simulink model "KF_3_gdl_AHRS_Dataset2"  (R2020b)
settings: Solver=FixedStepAuto  StartTime=0.0  StopTime=1000  FixedStep=1/200  RelTol=1e-3
values from neighbouring files (symbols this model uses):
  BARO_cov = single(1.7)/2    [init_1gdl.m]    (also in init_3_gdl_AHRS_fb.m = single(1.7)/5; init_3gdl.m; init_dati_veri.m = single(1.7)/5)
  BARO_cov_old = single(1.7)/2    [init_1gdl.m]    (also in init_3_gdl_AHRS_fb.m; init_3gdl.m; init_dati_veri.m)
  bj_x = 0.4    [init_3_gdl_AHRS_fb.m]
  bj_y = 0.9    [init_3_gdl_AHRS_fb.m]
  bj_z = 0.5    [init_3_gdl_AHRS_fb.m]
  bjy = bj_y - 0.1    (= 0.8)    [init_3_gdl_AHRS_fb.m]
  filter_pos = tf(1,[1 1])    [init_1gdl.m]    (also in init_3_gdl_AHRS_fb.m; init_3gdl.m; init_dati_veri.m)
  filter_pos_Z = tf(1,[0.5 1])    [init_3_gdl_AHRS_fb.m]    (also in init_3gdl.m; init_dati_veri.m)
  g_ned = [0; 0; -9.81]    [init_3_gdl_AHRS_fb.m]    (also in init_dati_veri.m)
  GPS_cov = single([1*2, 1])/2    [init_1gdl.m]    (also in init_3_gdl_AHRS_fb.m = single([0.1*50, 0.1*50, 200*5, 200*5, 0.36])/2; init_3gdl.m = single([1*2, 1*2, 1, 1, 0.36])/2; init_dati_veri.m = single([0.1, 0.1, 200*5, 200*5, 0.36])/2)
  GPS_cov_old = single([0.1, 0.1, 200, 200, 0.36])/2    [init_1gdl.m]    (also in init_3_gdl_AHRS_fb.m = single([0.1, 0.1, 200, 200, 0.36]/2); init_3gdl.m; init_dati_veri.m = single([0.1, 0.1, 200, 200, 0.36]/2))
  IMU_cov = single(15*0.07)/2    [init_1gdl.m]    (also in init_3_gdl_AHRS_fb.m = single([15*[0.07*50, 0.07*50] 15*50*0.09])/2; init_3gdl.m = single([15*[0.07, 0.07] 10*0.09])/2; init_dati_veri.m = single([15*[0.07*5, 0.07*5] 15*50*0.09])/2)
  IMU_cov_old = single([15*[0.07, 0.07] 10*0.09])/2    [init_1gdl.m]    (also in init_3_gdl_AHRS_fb.m = single([15*[0.07, 0.07] 10*0.09]/2); init_3gdl.m; init_dati_veri.m = single([15*[0.07, 0.07] 10*0.09]/2))
  Q = single(diag([1e-2, 1e-6, 1e-4, 1e-12]))*2    [init_1gdl.m]    (also in init_3_gdl_AHRS_fb.m = single(diag([px,vx,ax,py,vy,ay,pz,vz,az,bx,by,bz]))*2; init_3gdl.m = single(diag([px,vx,ax,py,vy,ay,pz,vz,az,bx,by,bz]))*2; init_dati_veri.m = single(diag([px,vx,ax,py,vy,ay,pz,vz,az,bx,by,bz]))*2)
  Q_old = single(diag([1e-8, 1e-1, 1e-2, 1e-8, 1e-1, 1e-2, 1e-5, 1e-4, 0.010]))*2    [init_1gdl.m]    (also in init_3_gdl_AHRS_fb.m; init_3gdl.m; init_dati_veri.m)
  ST = 1/200    (= 0.005)    [init_1gdl.m]    (also in init_3_gdl_AHRS_fb.m; init_3gdl.m; init_dati_veri.m)
  T_50 = 1/50    (= 0.02)    [init_1gdl.m]    (also in init_3_gdl_AHRS_fb.m; init_3gdl.m; init_dati_veri.m)
  var_giroscopio = [(deg2rad(0.16))^2;(deg2rad(0.16))^2;(deg2rad(0.16))^2]    [init_3_gdl_AHRS_fb.m]    (also in init_dati_veri.m)
  var_p_x = 2    [init_3_gdl_AHRS_fb.m]    (also in init_3gdl.m = 1; init_dati_veri.m)
  var_p_y = 2    [init_3_gdl_AHRS_fb.m]    (also in init_3gdl.m = 1; init_dati_veri.m)
  var_p_z = 0.30    (= 0.3)    [init_3_gdl_AHRS_fb.m]    (also in init_3gdl.m = 0.15; init_dati_veri.m)
  var_v_x = 0.60    (= 0.6)    [init_3_gdl_AHRS_fb.m]    (also in init_3gdl.m = 0.3; init_dati_veri.m)
  var_v_y = 0.32    [init_3_gdl_AHRS_fb.m]    (also in init_3gdl.m = 0.16; init_dati_veri.m)
  var_v_z = 0.60    (= 0.6)    [init_3_gdl_AHRS_fb.m]    (also in init_3gdl.m = 0.3; init_dati_veri.m)
undefined symbols (not defined in the file or in its folder): DiscIntNeverNeededParam
libraries: simulink x33, cstblocks x9
(part 1 of 4)
settings Model: Creator=chiara-s  LastModifiedBy=chiara-s

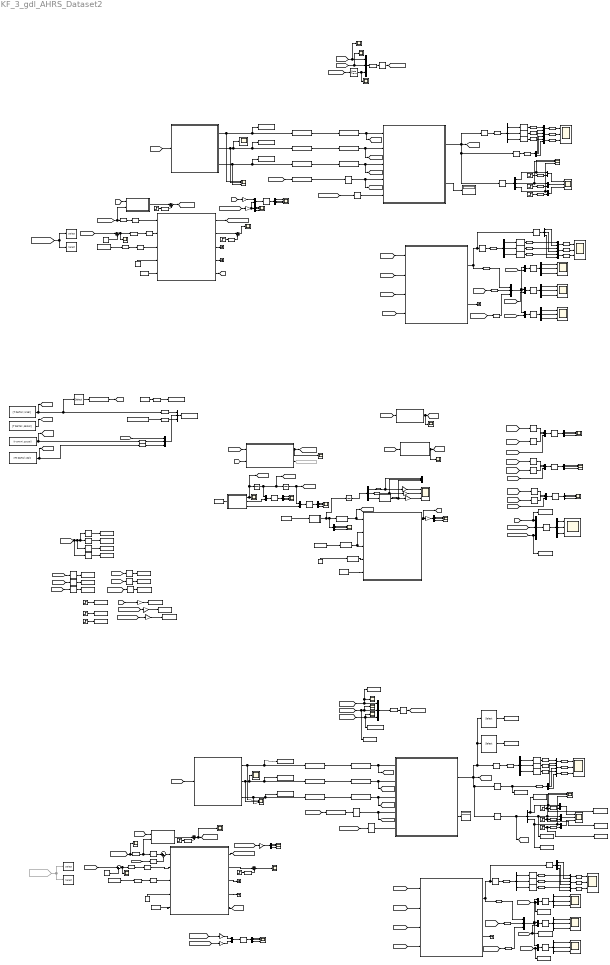
== system KF_3_gdl_AHRS_Dataset2 ==
  note: confronto filtro con feedback e filtro senza
  note: NO BIAS FEEDBACK
  note: AHRS CON FEEDBACK BIAS
  note: misurement DATA (già in NED)
  note: TAKE DATA
  note: inertial data
  note: KF_a_bordo_DATA
  note: FLAGS
  ACC : Scope  NumInputPorts=3
  ACC confronto : Scope  NumInputPorts=3
  ACC1 : Scope  NumInputPorts=3
  ACC_AHRS_NED1 : Scope
  ACC_DOPO_AHRS_NED COMPENSATO DI GRAVITA' : Scope
  ACC_DOPO_AHRS_NED COMPENSATO DI GRAVITA'1 : Scope
  CONFRONTO BIAS : Scope  NumInputPorts=3
  CONFRONTO BIAS1 : Scope  NumInputPorts=3
  Cast To Single{,1..5} (6 alike) : DataTypeConversion  OutDataTypeStr=single
  Confronto RPY_conRPY_feedback : Scope  NumInputPorts=3
  Constant : Constant  Value=[0;0;0]  VectorParams1D=off
  Constant1 : Constant  Value=[0;0;0]
  DATASET NOSTRO1 : MATLAB Function  TreatAsAtomicUnit=on
  Data Type Conversion{1..51,53,67..75,77..89} (74 alike) : DataTypeConversion  OutDataTypeStr=single
  Demux{,1..2,4..6,10..12,16,21..23,31,36} (15 alike) : Demux  Outputs=3
  Demux{13..14,19..20} (4 alike) : Demux  Outputs=[2 2 2]
  Demux{3,15,17..18} (4 alike) : Demux  Outputs=[3 3 3]
  Demux{7..9,37..39} (6 alike) : Demux  Outputs=[4 4 4]
  Digital Clock : DigitalClock  SampleTime=0.005
  Digital Clock1 : DigitalClock  SampleTime=0.02
  Digital Clock2 : DigitalClock  SampleTime=1/200
  Discrete Derivative{,1..11} (12 alike) : simulink/Discrete/Discrete Derivative  gainval=1.0  ICPrevScaledInput=0.0  OutMin=[]  OutMax=[]  OutDataType=fixdt(1, 16)  OutScaling=2^-10  DoSatur=off
  Discrete-Time Integrator : DiscreteIntegrator  SampleTime=-1  ICPrevOutput=DiscIntNeverNeededParam  ICPrevScaledInput=DiscIntNeverNeededParam
  Discrete-Time Integrator1 : DiscreteIntegrator  SampleTime=-1  ICPrevOutput=DiscIntNeverNeededParam  ICPrevScaledInput=DiscIntNeverNeededParam
  Discrete-Time Integrator2 : DiscreteIntegrator  SampleTime=-1  ICPrevOutput=DiscIntNeverNeededParam  ICPrevScaledInput=DiscIntNeverNeededParam
  Display : Display
  Display1 : Display
  Dpos VS vel_stima{,1..3} (4 alike) : Scope  NumInputPorts=3
  FLAG : Scope  NumInputPorts=3
  FLAG1 : Scope  NumInputPorts=3
  Flag computation : MATLAB Function  TreatAsAtomicUnit=on
  Flag computation1 : MATLAB Function  TreatAsAtomicUnit=on
  From73 : From  Commented=on  GotoTag=inertial_data
  Gain{,1..8,18..20} (12 alike) : Gain  Gain=180/pi
  Goto11 : Goto  Commented=on  GotoTag=accelorometro_vero
  MATLAB Function : MATLAB Function  TreatAsAtomicUnit=on
  MATLAB Function1 : MATLAB Function  TreatAsAtomicUnit=on
  MATLAB Function2 : MATLAB Function  TreatAsAtomicUnit=on
  MATLAB Function3 : MATLAB Function  TreatAsAtomicUnit=on
  MPU AHRS1 : Subsystem
  MPU AHRS3 : Subsystem
  MPU AHRS4 : Subsystem
  Mux{,1..5,8,11,13..19,24..25,27,37,39..43,46,56,63..64} (28 alike) : Mux  Inputs=2
  Mux{6..7,9..10,12,20..23,26,67} (11 alike) : Mux  Inputs=3
  Navigation Filter SINGLE 50 Hz NOSTRO : MATLAB Function  TreatAsAtomicUnit=on  mask{Q=Q, GPS_cov=GPS_cov, IMU_cov=IMU_cov, BARO_cov=BARO_cov}
      mask prompts: Q "Q matrix"; GPS_cov "R matrix - GPS covariance [px py vx vy vz]"; IMU_cov "R matrix - IMU covariance [ax ay az]"; BARO_cov "R matrix - BARO covariance"
  Navigation Filter SINGLE 50 Hz NOSTRO1 : MATLAB Function  TreatAsAtomicUnit=on  mask{Q=Q, GPS_cov=GPS_cov, IMU_cov=IMU_cov, BARO_cov=BARO_cov}
      mask prompts: Q "Q matrix"; GPS_cov "R matrix - GPS covariance [px py vx vy vz]"; IMU_cov "R matrix - IMU covariance [ax ay az]"; BARO_cov "R matrix - BARO covariance"
  Navigation Filter SINGLE 50 Hz1 : MATLAB Function  TreatAsAtomicUnit=on  mask{Q=Q_old, GPS_cov=GPS_cov, IMU_cov=IMU_cov, BARO_cov=BARO_cov}
      mask prompts: Q "Q matrix"; GPS_cov "R matrix - GPS covariance [px py vx vy vz]"; IMU_cov "R matrix - IMU covariance [ax ay az]"; BARO_cov "R matrix - BARO covariance"
  Navigation Filter SINGLE 50 Hz2 : MATLAB Function  TreatAsAtomicUnit=on  mask{Q=Q_old, GPS_cov=GPS_cov_old, IMU_cov=IMU_cov_old, BARO_cov=BARO_cov_old}
      mask prompts: Q "Q matrix"; GPS_cov "R matrix - GPS covariance [px py vx vy vz]"; IMU_cov "R matrix - IMU covariance [ax ay az]"; BARO_cov "R matrix - BARO covariance"
  POS confronto : Scope  NumInputPorts=3
  POSITION : Scope  NumInputPorts=3
  POSITION1 : Scope  NumInputPorts=3
  RPY : Scope  NumInputPorts=3
  RPY degree : Scope  NumInputPorts=3
  RPY degree2 : Scope  NumInputPorts=3
  RPY1 : Scope  NumInputPorts=3
  Random Number : RandomNumber  Variance=var_giroscopio  Seed=[1; 5; 3]  SampleTime=1/200  VectorParams1D=off
  Random Number1 : RandomNumber  Variance=var_giroscopio  Seed=[1; 5; 3]  SampleTime=1/200  VectorParams1D=off
  Rate Transition{1,3..4,11,15,30..35} (11 alike) : RateTransition  OutPortSampleTime=1/50
  Rate Transition{5..8,16..18} (7 alike) : RateTransition  OutPortSampleTime=1/200
  Scope{,4..6} (4 alike) : Scope  NumInputPorts=3
  Scope1 : Scope
  Scope2 : Scope
  Scope7 : Scope
  Selector : Selector  InputPortWidth=12  IndexOptions=Index vector (dialog)  Indices=[10 11 12]  OutputSizes=1
  Selector{1,5,19..20,33,47} (6 alike) : Selector  InputPortWidth=12  IndexOptions=Index vector (dialog)  Indices=[1 4 7]  OutputSizes=1
  Selector10 : Selector  InputPortWidth=30+3  IndexOptions=Index vector (dialog)  Indices=[2 11 23 31 5 14 26 32 8 17 29 33]  OutputSizes=1
  Selector11 : Selector  InputPortWidth=30+3  IndexOptions=Index vector (dialog)  Indices=[3 12 24 31 6 15 27 32 9 18 30 33]  OutputSizes=1
  Selector12 : Selector  InputPortWidth=9  IndexOptions=Index vector (dialog)  Indices=[1 4 7]  OutputSizes=1
  Selector13 : Selector  InputPortWidth=30+3  IndexOptions=Index vector (dialog)  Indices=[1 10 22 31 4 13 25 32 7 16 28 33]  OutputSizes=1
  Selector14 : Selector  InputPortWidth=9  IndexOptions=Index vector (dialog)  Indices=[2 5 8]  OutputSizes=1
  Selector15 : Selector  InputPortWidth=9  IndexOptions=Index vector (dialog)  Indices=[2 5 8]  OutputSizes=1
  Selector{16..17,28,30} (4 alike) : Selector  InputPortWidth=6  IndexOptions=Index vector (dialog)  Indices=[1 4 2 5 3 6]  OutputSizes=1
  Selector{2,18,21,24,27,31} (6 alike) : Selector  InputPortWidth=9  IndexOptions=Index vector (dialog)  Indices=[1 4 7 2 5 8 3 6 9]  OutputSizes=1
  Selector{3,22..23,29,46} (5 alike) : Selector  InputPortWidth=12  IndexOptions=Index vector (dialog)  Indices=[2 5 8]  OutputSizes=1
  Selector{25..26,32,48} (4 alike) : Selector  InputPortWidth=12  IndexOptions=Index vector (dialog)  Indices=[3 6 9]  OutputSizes=1
  Selector4 : Selector  InputPortWidth=12  IndexOptions=Index vector (dialog)  Indices=[10 11 12]  OutputSizes=1
  Selector49 : Selector  InputPortWidth=12  IndexOptions=Index vector (dialog)  Indices=[10 11 12]  OutputSizes=1
  Selector6 : Selector  InputPortWidth=30+3  IndexOptions=Index vector (dialog)  Indices=[2 11 23 31 5 14 26 32 8 17 29 33]  OutputSizes=1
  Selector7 : Selector  InputPortWidth=30+3  IndexOptions=Index vector (dialog)  Indices=[3 12 24 31 6 15 27 32 9 18 30 33]  OutputSizes=1
  Selector8 : Selector  InputPortWidth=9  IndexOptions=Index vector (dialog)  Indices=[1 4 7]  OutputSizes=1
  Selector9 : Selector  InputPortWidth=30+3  IndexOptions=Index vector (dialog)  Indices=[1 10 22 31 4 13 25 32 7 16 28 33]  OutputSizes=1
  Subsystem : Subsystem
  Subsystem1 : Subsystem
  Subsystem2 : Subsystem
  Sum{,1,3..6} (6 alike) : Sum  Inputs=|++
  Sum2 : Sum  Inputs=|+-
  Terminator{,1..5} (6 alike) : Terminator
  To Workspace : ToWorkspace  VariableName=pos_vera  SaveFormat=Timeseries  SampleTime=-1
  To Workspace1 : ToWorkspace  VariableName=vel_vera  SaveFormat=Timeseries  SampleTime=-1
  To Workspace10 : ToWorkspace  VariableName=baro_fix_flag  SampleTime=-1
  To Workspace11 : ToWorkspace  VariableName=acc_misura  SaveFormat=Timeseries  SampleTime=-1
  To Workspace12 : ToWorkspace  VariableName=vel_misura  SaveFormat=Timeseries  SampleTime=-1
  To Workspace13 : ToWorkspace  VariableName=pos_misura  SaveFormat=Timeseries  SampleTime=-1
  To Workspace14 : ToWorkspace  VariableName=bias_x  SaveFormat=Timeseries  SampleTime=-1
  To Workspace15 : ToWorkspace  VariableName=bias_y  SaveFormat=Timeseries  SampleTime=-1
  To Workspace16 : ToWorkspace  VariableName=bias_z  SaveFormat=Timeseries  SampleTime=-1
  To Workspace17 : ToWorkspace  VariableName=vel_stima  SaveFormat=Timeseries  SampleTime=-1
  To Workspace18 : ToWorkspace  VariableName=acc_stima  SaveFormat=Timeseries  SampleTime=-1
  To Workspace19 : ToWorkspace  VariableName=rpy_vera  SaveFormat=Timeseries  SampleTime=-1
  To Workspace2 : ToWorkspace  VariableName=acc_vera  SaveFormat=Timeseries  SampleTime=-1
  To Workspace20 : ToWorkspace  VariableName=rpy_feedback  SaveFormat=Timeseries  SampleTime=-1
  To Workspace21 : ToWorkspace  VariableName=pos_stima  SaveFormat=Timeseries  SampleTime=-1
  To Workspace22 : ToWorkspace  VariableName=bx_cost  SaveFormat=Timeseries  SampleTime=-1
  To Workspace23 : ToWorkspace  VariableName=by_cost  SaveFormat=Timeseries  SampleTime=-1
  To Workspace24 : ToWorkspace  VariableName=bz_cost  SaveFormat=Timeseries  SampleTime=-1
  To Workspace3 : ToWorkspace  VariableName=gps_fix_flag  SampleTime=-1
  To Workspace4 : ToWorkspace  VariableName=init_flag  SampleTime=-1
  To Workspace5 : ToWorkspace  VariableName=DATA_1  SampleTime=-1
  To Workspace6 : ToWorkspace  VariableName=T_1  SampleTime=-1
  To Workspace7 : ToWorkspace  VariableName=gps_fix_flag1  SampleTime=-1
  To Workspace73 : ToWorkspace  VariableName=pos_misura1  SaveFormat=Timeseries  SampleTime=-1
  To Workspace74 : ToWorkspace  VariableName=vel_misura1  SaveFormat=Timeseries  SampleTime=-1
  To Workspace75 : ToWorkspace  VariableName=pos_vera1  SaveFormat=Timeseries  SampleTime=-1
  To Workspace76 : ToWorkspace  VariableName=vel_vera1  SaveFormat=Timeseries  SampleTime=-1
  To Workspace77 : ToWorkspace  VariableName=acc_vera1  SaveFormat=Timeseries  SampleTime=-1
  To Workspace78 : ToWorkspace  VariableName=pos_stima1  SaveFormat=Timeseries  SampleTime=-1
  To Workspace79 : ToWorkspace  VariableName=vel_stima1  SaveFormat=Timeseries  SampleTime=-1
  To Workspace8 : ToWorkspace  VariableName=init_flag1  SampleTime=-1
  To Workspace80 : ToWorkspace  VariableName=acc_stima1  SaveFormat=Timeseries  SampleTime=-1
  To Workspace81 : ToWorkspace  VariableName=bias_stima1  SaveFormat=Timeseries  SampleTime=-1
  To Workspace82 : ToWorkspace  VariableName=bx_vero  SaveFormat=Timeseries  SampleTime=-1
  To Workspace83 : ToWorkspace  VariableName=by_vero  SaveFormat=Timeseries  SampleTime=-1
  To Workspace84 : ToWorkspace  VariableName=acc_misura1  SaveFormat=Timeseries  SampleTime=-1
  To Workspace85 : ToWorkspace  VariableName=bz_vero  SaveFormat=Timeseries  SampleTime=-1
  To Workspace86 : ToWorkspace  VariableName=rpy_ideali  SaveFormat=Timeseries  SampleTime=-1
  To Workspace87 : ToWorkspace  VariableName=rpy  SaveFormat=Timeseries  SampleTime=-1
  To Workspace88 : ToWorkspace  VariableName=rpy_fb  SaveFormat=Timeseries  SampleTime=-1
  To Workspace9 : ToWorkspace  VariableName=baro_fix_flag1  SampleTime=-1
  VEL confronto : Scope  NumInputPorts=3
  VELOCITY : Scope  NumInputPorts=3
  VELOCITY1 : Scope  NumInputPorts=3
  acc : Scope
  acc_body_g : Scope
  acccc2 : Scope
  acccc3 : Scope
  angular rate : Scope  NumInputPorts=3
  b_x : Step  Time=0  After=bj_x  SampleTime=T_50
  b_x1 : Step  Time=0  After=bj_x  SampleTime=T_50
  b_x5 : Step  Time=0  After=bj_x  SampleTime=T_50
  b_y : Step  Time=0  After=bj_y  SampleTime=T_50
  b_y1 : Step  Time=0  After=bjy  SampleTime=T_50
  b_y5 : Step  Time=0  After=bjy  SampleTime=T_50
  b_z : Step  Time=0  After=bj_z  SampleTime=T_50
  b_z1 : Step  Time=0  After=bj_z  SampleTime=T_50
  b_z5 : Step  Time=0  After=bj_z  SampleTime=T_50
  disable1 : Constant  Value=0
  disable2 : Constant  Value=0
  disable3 : Constant  Value=0
  dummy VICON angles 1 : Constant  Value=[0; 0; 0]  OutDataTypeStr=single
  dummy VICON angles 2 : Constant  Value=[0; 0; 0]  OutDataTypeStr=single
  dummy VICON angles 3 : Constant  Value=[0; 0; 0]  OutDataTypeStr=single
  get MAG1 : Selector  InputPortWidth=15  IndexOptions=Index vector (dialog)  Indices=[11:13]  OutputSizes=1
  get MAG2 : Selector  InputPortWidth=15  IndexOptions=Index vector (dialog)  Indices=[5:7]  OutputSizes=1
  get MAG3 : Selector  InputPortWidth=15  IndexOptions=Index vector (dialog)  Indices=[11:13]  OutputSizes=1
  get OMEGA4 : Selector  InputPortWidth=15  IndexOptions=Index vector (dialog)  Indices=[5:7]  OutputSizes=1
  get RPY1 : Selector  InputPortWidth=15  IndexOptions=Index vector (dialog)  Indices=[2:4]  OutputSizes=1
  get flags 1 : FromWorkspace  VariableName=[Tt DATA(:,34)]  SampleTime=0.02  OutputAfterFinalValue=Holding final value
  "get measurement data " : FromWorkspace  VariableName=[T DATA(:,25:33)]  SampleTime=0.02  OutputAfterFinalValue=Holding final value
  get navdata(KF) : FromWorkspace  VariableName=[T DATA(:,16:24)]  SampleTime=0.02  OutputAfterFinalValue=Holding final value
  get navdata4 : FromWorkspace  VariableName=[T DATA(:,1:15)]  SampleTime=0.02  Interpolate=off  OutputAfterFinalValue=Holding final value
  get navdata5 : FromWorkspace  VariableName=[T DATA(:,35:40)]  SampleTime=0.02  Interpolate=off  OutputAfterFinalValue=Holding final value
  gps fix1 : Scope
  gps fix2 : Scope
  gravity : Step  Time=0  After=[0; 0; 9.81]  SampleTime=1/200
  gravity1 : Step  Time=11.02  After=[0; 0; 9.81]  SampleTime=1/200
  gravity2 : Step  Time=0  After=[0; 0; 9.81]  SampleTime=1/200
  gravity3 : Step  Time=0  After=[0; 0; 9.81]  SampleTime=1/200
  mag : Constant  Value=[0;0;0]
  pos : Scope  NumInputPorts=3
  pos_misura : Scope
  poss2 : Scope
  poss3 : Scope
  vel : Scope  NumInputPorts=3
  vel_misura : Scope
  velll2 : Scope
  velll3 : Scope
  wires:
  Data Type Conversion19/1 -> To Workspace6/1
  Data Type Conversion25/1 -> Data Type Conversion26/1
  Data Type Conversion17/1 -> Mux10/1
  Data Type Conversion29/1 -> Rate Transition4/1
  [x_out_filter] -> Mux12/1
  Data Type Conversion28/1 -> [flag_baro], Navigation Filter SINGLE 50 Hz NOSTRO/3(flagBARO)
  Navigation Filter SINGLE 50 Hz NOSTRO/1(xout) -> Selector/1, Selector3/1, [x_out_filter], Selector1/1
  get navdata4/1 -> get RPY1/1, Data Type Conversion17/1, [inertial_data]
  Data Type Conversion18/1 -> Mux12/2
  Data Type Conversion24/1 -> [flag_init_ok], Navigation Filter SINGLE 50 Hz NOSTRO/1(flagINITOK)
  Mux12/1 -> Mux10/2
  Data Type Conversion22/1 -> Mux10/3
  Data Type Conversion27/1 -> Data Type Conversion28/1
  Flag computation/1(init) -> To Workspace8/1, Data Type Conversion23/1, FLAG/1
  Data Type Conversion21/1 -> Mux12/3
  get navdata5/1 -> Data Type Conversion22/1
  Digital Clock1/1 -> Data Type Conversion19/1
  Navigation Filter SINGLE 50 Hz NOSTRO/2(Pout) -> Display/1
  Data Type Conversion26/1 -> [flag_GPS], Navigation Filter SINGLE 50 Hz NOSTRO/2(flagGPS)
  get flags 1/1 -> [flag_data], Data Type Conversion21/1
  Rate Transition4/1 -> [measure], Navigation Filter SINGLE 50 Hz NOSTRO/4(measure)
  Data Type Conversion23/1 -> Data Type Conversion24/1
  Flag computation/2(gps) -> To Workspace7/1, Data Type Conversion25/1, gps fix1/1, FLAG/2
  "get measurement data "/1 -> [measurements], Data Type Conversion18/1
  get navdata(KF)/1 -> [nav_data_KF]
  Flag computation/3(baro) -> To Workspace9/1, Data Type Conversion27/1, FLAG/3
  Mux10/1 -> To Workspace5/1
  Selector1/1 -> Data Type Conversion13/1
  [dataset_AHRS] -> Data Type Conversion29/1
  Selector/1 -> Demux1/1
  b_x/1 -> Data Type Conversion3/1
  Mux/1 -> CONFRONTO BIAS/1
  Demux1/2 -> Scope/2, Mux2/1
  b_y/1 -> Data Type Conversion2/1
  Mux2/1 -> CONFRONTO BIAS/2
  b_z/1 -> Data Type Conversion1/1
  Demux1/3 -> Scope/3, Mux1/1
  Mux1/1 -> CONFRONTO BIAS/3
  Data Type Conversion1/1 -> Mux1/2
  Data Type Conversion2/1 -> Mux2/2
  Demux/1 -> Discrete Derivative/1
  Demux/2 -> Discrete Derivative2/1
  Demux/3 -> Discrete Derivative1/1
  Selector3/1 -> Data Type Conversion14/1
  Mux3/1 -> Data Type Conversion32/1
  Demux2/1 -> Mux3/2
  Mux4/1 -> Data Type Conversion31/1
  Demux2/2 -> Mux4/2
  Mux5/1 -> Data Type Conversion30/1
  Demux2/3 -> Mux5/2
  Data Type Conversion13/1 -> Demux/1
  Data Type Conversion14/1 -> Demux2/1
  Discrete Derivative1/1 -> Data Type Conversion15/1
  Data Type Conversion15/1 -> Mux5/1
  Discrete Derivative2/1 -> Data Type Conversion16/1
  Data Type Conversion16/1 -> Mux4/1
  Discrete Derivative/1 -> Data Type Conversion20/1
  Data Type Conversion20/1 -> Mux3/1
  Data Type Conversion30/1 -> Dpos VS vel_stima/3
  Data Type Conversion31/1 -> Dpos VS vel_stima/2
  Data Type Conversion32/1 -> Dpos VS vel_stima/1
  Data Type Conversion3/1 -> Mux/2
  Demux1/1 -> Scope/1, Mux/1
  get RPY1/1 -> Data Type Conversion33/1
  Data Type Conversion33/1 -> [RPY]
  [RPY_AHRS] -> Rate Transition1/1
  Demux6/1 -> RPY degree/1
  Demux6/2 -> RPY degree/2
  Demux6/3 -> RPY degree/3
  [flag_init_ok] -> Navigation Filter SINGLE 50 Hz1/1(flagINITOK)
  [flag_GPS] -> Navigation Filter SINGLE 50 Hz1/2(flagGPS)
  [flag_baro] -> Navigation Filter SINGLE 50 Hz1/3(flagBARO)
  [measure] -> Navigation Filter SINGLE 50 Hz1/4(measure)
  Navigation Filter SINGLE 50 Hz1/2(Pout) -> Terminator/1
  Navigation Filter SINGLE 50 Hz1/1(xout) -> Data Type Conversion34/1, Selector14/1, Selector12/1
  [x_out_filter] -> Data Type Conversion35/1
  [dataset_AHRS] -> Data Type Conversion36/1
  Data Type Conversion34/1 -> Mux9/1
  Data Type Conversion35/1 -> Mux9/2
  Data Type Conversion36/1 -> Mux9/3
  Selector13/1 -> Demux7/1
  Demux7/1 -> POSITION/1
  Demux7/2 -> POSITION/2
  Demux7/3 -> POSITION/3
  Selector10/1 -> Demux8/1
  Selector11/1 -> Demux9/1
  Demux9/1 -> ACC/1
  Demux9/2 -> ACC/2
  Demux9/3 -> ACC/3
  Demux8/1 -> VELOCITY/1
  Demux8/2 -> VELOCITY/2
  Demux8/3 -> VELOCITY/3
  Discrete Derivative4/1 -> Data Type Conversion38/1
  Data Type Conversion37/1 -> Demux10/1
  Demux10/1 -> Discrete Derivative3/1
  Discrete Derivative3/1 -> Data Type Conversion40/1
  Discrete Derivative5/1 -> Data Type Conversion39/1
  Demux10/2 -> Discrete Derivative5/1
  Demux10/3 -> Discrete Derivative4/1
  Selector12/1 -> Data Type Conversion37/1
  Data Type Conversion40/1 -> Mux11/1
  Mux14/1 -> Data Type Conversion41/1
  Data Type Conversion39/1 -> Mux13/1
  Data Type Conversion41/1 -> Dpos VS vel_stima1/3
  Data Type Conversion38/1 -> Mux14/1
  Mux13/1 -> Data Type Conversion42/1
  Data Type Conversion42/1 -> Dpos VS vel_stima1/2
  Mux11/1 -> Data Type Conversion43/1
  Data Type Conversion43/1 -> Dpos VS vel_stima1/1
  Selector14/1 -> Demux11/1
  Demux11/1 -> Mux11/2
  Demux11/2 -> Mux13/2
  Demux11/3 -> Mux14/2
  Mux15/1 -> Selector13/1
  Mux16/1 -> Selector10/1
  Mux17/1 -> Selector11/1
  Mux9/1 -> Mux17/1, Mux15/1, Mux16/1
  [pos_ned_vera] -> Mux15/2
  [vel_ned_vera] -> Mux16/2
  [acc_ned_vera] -> Mux17/2
  disable1/1 -> MPU AHRS1/4(vicon_enable)
  Data Type Conversion45/1 -> Rate Transition6/1
  Rate Transition6/1 -> MPU AHRS1/3(MAG)
  Data Type Conversion44/1 -> Rate Transition5/1
  Rate Transition7/1 -> MPU AHRS1/2(PQR)
  dummy VICON angles 1/1 -> MPU AHRS1/5(Vicon_ori)
  MPU AHRS1/1(RPY_MPU) -> [RPY_AHRS]
  MPU AHRS1/4(debiased PQR) -> Terminator1/1
  MPU AHRS1/3(filter running) -> Terminator2/1
  [inertial_data] -> get MAG1/1, get MAG2/1
  Data Type Conversion46/1 -> Rate Transition7/1
  [RPY_AHRS] -> Gain/1
  Rate Transition1/1 -> Navigation Filter SINGLE 50 Hz NOSTRO/5(euler_in)
  MPU AHRS1/5(Rt) -> [Rt]
  Rate Transition11/1 -> Navigation Filter SINGLE 50 Hz NOSTRO1/5(euler_in)
  Data Type Conversion8/1 -> Mux63/1
  Demux22/3 -> Discrete Derivative10/1
  Data Type Conversion69/1 -> Data Type Conversion70/1
  [RPY_AHRS_fd] -> Rate Transition11/1
  MPU AHRS4/5(Rt) -> [Rt_fd]
  Demux23/2 -> Mux39/2
  MPU AHRS4/2(ACC_NED) -> Sum3/1
  Flag computation1/1(init) -> FLAG1/1, To Workspace4/1, Data Type Conversion51/1
  Selector4/1 -> [bias_stima_fd], Demux16/1
  Mux37/1 -> Data Type Conversion86/1
  MPU AHRS4/4(debiased PQR) -> Terminator4/1
  MPU AHRS4/3(filter running) -> Terminator5/1
  Selector8/1 -> Data Type Conversion80/1
  Data Type Conversion84/1 -> Dpos VS vel_stima3/3
  Demux36/3 -> RPY degree2/3
  Demux39/1 -> ACC1/1
  Data Type Conversion48/1 -> Mux56/1
  Mux41/1 -> Selector9/1
  Mux39/1 -> Data Type Conversion85/1
  Selector9/1 -> Demux37/1
  Data Type Conversion5/1 -> Demux5/1
  Gain5/1 -> Demux36/1
  Flag computation1/2(gps) -> gps fix2/1, To Workspace3/1, Data Type Conversion67/1, FLAG1/2
  Selector7/1 -> Demux39/1
  Data Type Conversion78/1 -> Mux67/2
  Navigation Filter SINGLE 50 Hz NOSTRO1/2(Pout) -> Display1/1
  Mux56/1 -> Data Type Conversion75/1
  Mux63/1 -> Data Type Conversion74/1
  Data Type Conversion83/1 -> Mux37/1
  Discrete Derivative6/1 -> Data Type Conversion48/1
  [x_out_filter_fd] -> Data Type Conversion78/1
  From73/1 -> get MAG3/1, get OMEGA4/1
  Navigation Filter SINGLE 50 Hz2/2(Pout) -> Terminator3/1
  dummy VICON angles 2/1 -> MPU AHRS4/5(Vicon_ori)
  Mux67/1 -> Mux43/1, Mux41/1, Mux42/1
  Data Type Conversion89/1 -> Rate Transition18/1
  MPU AHRS4/1(RPY_MPU) -> [RPY_AHRS_fd]
  [RPY_AHRS_fd] -> Gain5/1
  Demux16/1 -> To Workspace14/1, Scope5/1, Mux8/1
  Demux37/3 -> POSITION1/3
  Mux43/1 -> Selector7/1
  disable2/1 -> MPU AHRS4/4(vicon_enable)
  Rate Transition17/1 -> MPU AHRS4/3(MAG)
  Rate Transition18/1 -> MPU AHRS4/2(PQR)
  Discrete Derivative11/1 -> Data Type Conversion82/1
  [pos_ned_vera] -> To Workspace/1, Mux41/2
  Data Type Conversion80/1 -> Demux22/1
  [flag_GPS_fd] -> Navigation Filter SINGLE 50 Hz2/2(flagGPS)
  Selector15/1 -> Demux23/1
  Mux46/1 -> CONFRONTO BIAS1/2
  Demux38/1 -> VELOCITY1/1
  Data Type Conversion85/1 -> Dpos VS vel_stima3/2
  Data Type Conversion74/1 -> Dpos VS vel_stima2/2
  Demux38/3 -> VELOCITY1/3
  Demux22/1 -> Discrete Derivative9/1
  Data Type Conversion82/1 -> Mux39/1
  Mux42/1 -> Selector6/1
  Discrete Derivative9/1 -> Data Type Conversion83/1
  Demux23/1 -> Mux37/2
  Rate Transition15/1 -> [measure_fd], Navigation Filter SINGLE 50 Hz NOSTRO1/4(measure)
  Demux22/2 -> Discrete Derivative11/1
  Data Type Conversion81/1 -> Mux40/1
  Discrete Derivative10/1 -> Data Type Conversion81/1
  Demux38/2 -> VELOCITY1/2
  Demux39/3 -> ACC1/3
  Demux39/2 -> ACC1/2
  Data Type Conversion67/1 -> Data Type Conversion68/1
  Discrete Derivative7/1 -> Data Type Conversion7/1
  Selector6/1 -> Demux38/1
  Demux37/2 -> POSITION1/2
  Data Type Conversion77/1 -> Mux67/1
  Data Type Conversion79/1 -> Mux67/3
  Demux36/2 -> RPY degree2/2
  Data Type Conversion75/1 -> Dpos VS vel_stima2/1
  Demux36/1 -> RPY degree2/1
  Selector29/1 -> To Workspace17/1, Data Type Conversion6/1
  Demux31/2 -> Mux63/2
  Demux31/3 -> Mux64/2
  b_z1/1 -> To Workspace24/1, Data Type Conversion4/1
  b_y1/1 -> To Workspace23/1, Data Type Conversion12/1
  Data Type Conversion12/1 -> Mux46/2
  Data Type Conversion4/1 -> Mux27/2
  [dataset_AHRS_fd] -> Data Type Conversion79/1
  Data Type Conversion70/1 -> [flag_baro_fd], Navigation Filter SINGLE 50 Hz NOSTRO1/3(flagBARO)
  Data Type Conversion7/1 -> Mux64/1
  Data Type Conversion68/1 -> [flag_GPS_fd], Navigation Filter SINGLE 50 Hz NOSTRO1/2(flagGPS)
  Data Type Conversion88/1 -> Rate Transition17/1
  Mux8/1 -> CONFRONTO BIAS1/1
  Data Type Conversion51/1 -> Data Type Conversion53/1
  Demux5/2 -> Discrete Derivative8/1
  Mux27/1 -> CONFRONTO BIAS1/3
  Data Type Conversion71/1 -> Rate Transition15/1
  Demux23/3 -> Mux40/2
  Flag computation1/3(baro) -> To Workspace10/1, Data Type Conversion69/1, FLAG1/3
  Mux64/1 -> Data Type Conversion73/1
  [dataset_AHRS_fd] -> Data Type Conversion71/1
  Data Type Conversion73/1 -> Dpos VS vel_stima2/3
  Data Type Conversion53/1 -> [flag_init_ok_fd], Navigation Filter SINGLE 50 Hz NOSTRO1/1(flagINITOK)
  Demux16/2 -> To Workspace15/1, Scope5/2, Mux46/1
  Data Type Conversion86/1 -> Dpos VS vel_stima3/1
  Demux31/1 -> Mux56/2
  [measure_fd] -> Navigation Filter SINGLE 50 Hz2/4(measure)
  Demux5/1 -> Discrete Derivative6/1
  Demux37/1 -> POSITION1/1
  Discrete Derivative8/1 -> Data Type Conversion8/1
  [vel_ned_vera] -> To Workspace1/1, Mux42/2
  [flag_init_ok_fd] -> Navigation Filter SINGLE 50 Hz2/1(flagINITOK)
  Demux5/3 -> Discrete Derivative7/1
  Demux16/3 -> Scope5/3, Mux27/1, To Workspace16/1
  Mux40/1 -> Data Type Conversion84/1
  Navigation Filter SINGLE 50 Hz NOSTRO1/1(xout) -> Selector4/1, Selector29/1, [x_out_filter_fd], Selector33/1, Selector32/1, Selector5/1
  Navigation Filter SINGLE 50 Hz2/1(xout) -> Data Type Conversion77/1, Selector15/1, Selector8/1
  Selector5/1 -> Data Type Conversion5/1
  b_x1/1 -> To Workspace22/1, Data Type Conversion72/1
  Data Type Conversion72/1 -> Mux8/2
  Data Type Conversion6/1 -> Demux31/1
  [flag_baro_fd] -> Navigation Filter SINGLE 50 Hz2/3(flagBARO)
  [flag_data] -> Flag computation/1(flags)
  [flag_data] -> Flag computation1/1(flags)
  [acc_g_sporca_body] -> Scope7/1, Data Type Conversion87/1
  Rate Transition5/1 -> MPU AHRS1/1(ACC)
  Subsystem/1(acc_sporca) -> [acc_g_sporca_body], acc_body_g/1
  [vel_ned_vera] -> Subsystem1/1(vel_ned_pulita)
  Subsystem1/1(vel_misura) -> vel_misura/1, [vel_misura]
  Subsystem2/1(pos_misura) -> pos_misura/1, [pos_misura]
  [pos_ned_vera] -> Subsystem2/1(pos_pulita)
  Data Type Conversion11/1 -> Selector31/1
  [vel_misura] -> velll2/1, Mux6/2
  [pos_misura] -> poss2/1, Mux6/1
  Selector31/1 -> [dataset_AHRS]
  Mux6/1 -> Data Type Conversion11/1
  Rate Transition3/1 -> acccc2/1, Mux6/3
  [acc_ned_AHRS] -> Rate Transition3/1
  [vel_misura] -> To Workspace12/1, Mux7/2, velll3/1
  Selector2/1 -> [dataset_AHRS_fd]
  [pos_misura] -> To Workspace13/1, poss3/1, Mux7/1
  Mux7/1 -> Data Type Conversion47/1
  [acc_ned_AHRS_fd] -> Mux7/3, acccc3/1, To Workspace11/1
  Data Type Conversion47/1 -> Selector2/1
  Sum/1 -> ACC_AHRS_NED1/1
  MPU AHRS1/2(ACC_NED) -> Sum/1
  gravity/1 -> Data Type Conversion9/1
  Data Type Conversion9/1 -> Sum/2
  Subsystem/2(acceleromentro_vero) -> Goto11/1
  [acc_g_sporca_body] -> MATLAB Function/2(acc_body_sporca), Data Type Conversion44/1
  Digital Clock/1 -> MATLAB Function2/1(time)
  Demux4/1 -> angular rate/1
  Demux4/2 -> angular rate/2
  Demux4/3 -> angular rate/3
  disable3/1 -> Cast To Single1/1
  dummy VICON angles 3/1 -> MPU AHRS3/5(Vicon_ori)
  Constant/1 -> Cast To Single2/1
  MPU AHRS3/1(RPY_MPU) -> [prova], Gain1/1
  Demux12/1 -> RPY/1
  Demux12/2 -> RPY/2
  Demux12/3 -> RPY/3
  Cast To Single1/1 -> MPU AHRS3/4(vicon_enable)
  Cast To Single2/1 -> MPU AHRS3/2(MAG), MPU AHRS3/3(ACC)
  Cast To Single3/1 -> [PQR_veri], MPU AHRS3/1(PQR)
  Gain1/1 -> Demux12/1
  [prova] -> Gain2/1
  Gain2/1 -> Mux18/1
  Gain/1 -> Mux18/2, Demux6/1
  Mux18/1 -> Selector16/1
  Selector16/1 -> Demux13/1
  Demux13/2 -> Scope4/2
  Demux13/1 -> Scope4/1
  Demux13/3 -> Scope4/3
  [acc_ned_vera] -> To Workspace2/1, Mux43/2
  Data Type Conversion10/1 -> Sum3/2
  gravity1/1 -> Data Type Conversion10/1
  Sum3/1 -> ACC_DOPO_AHRS_NED COMPENSATO DI GRAVITA'/1
  Gain3/1 -> Mux19/1
  Demux14/3 -> Scope6/3
  Selector17/1 -> Demux14/1
  [prova] -> Gain3/1
  Demux14/1 -> Scope6/1
  Demux14/2 -> Scope6/2
  Mux19/1 -> Selector17/1
  [RPY_AHRS_fd] -> Gain4/1
  Gain4/1 -> Mux19/2
  Constant1/1 -> Data Type Conversion88/1
  mag/1 -> Data Type Conversion45/1
  [prova] -> Subsystem/2(rpy_int)
  MATLAB Function2/1(omega) -> Discrete-Time Integrator2/1, Cast To Single3/1, Demux4/1
  [x_out_filter] -> Selector19/1
  [x_out_filter_fd] -> Selector20/1
  Selector19/1 -> Mux21/1
  Selector20/1 -> Mux21/2
  Mux21/1 -> Selector21/1
  Selector21/1 -> Demux15/1
  [pos_ned_vera] -> Mux21/3
  Demux15/1 -> POS confronto/1
  Selector24/1 -> Demux17/1
  [x_out_filter_fd] -> Selector23/1
  Demux17/1 -> VEL confronto/1
  [x_out_filter] -> Selector22/1
  Demux17/2 -> VEL confronto/2
  Demux17/3 -> VEL confronto/3
  Mux22/1 -> Selector24/1
  Selector23/1 -> Mux22/2
  Selector22/1 -> Mux22/1
  [vel_ned_vera] -> Mux22/3
  Selector25/1 -> Mux23/1
  Selector26/1 -> Mux23/2
  [x_out_filter] -> Selector25/1
  Selector27/1 -> Demux18/1
  [x_out_filter_fd] -> Selector26/1
  Mux23/1 -> Selector27/1
  [acc_ned_vera] -> Mux23/3
  Demux3/3 -> Confronto RPY_conRPY_feedback/3
  [RPY_AHRS_fd] -> To Workspace20/1, Mux20/3
  [RPY_AHRS] -> Mux20/2
  Mux20/1 -> Selector18/1
  Demux3/2 -> Confronto RPY_conRPY_feedback/2
  Demux3/1 -> Confronto RPY_conRPY_feedback/1
  Selector18/1 -> Demux3/1
  [prova] -> To Workspace19/1, Mux20/1
  Demux15/2 -> POS confronto/2
  Demux15/3 -> POS confronto/3
  Demux18/1 -> ACC confronto/1
  Demux18/2 -> ACC confronto/2
  Demux18/3 -> ACC confronto/3
  Demux19/3 -> vel/3
  Selector30/1 -> Demux20/1
  Mux24/1 -> Selector28/1
  Demux19/2 -> vel/2
  Discrete-Time Integrator1/1 -> [pos_ned_vera], Mux25/1
  Demux20/3 -> pos/3
  Demux20/1 -> pos/1
  Discrete-Time Integrator/1 -> Mux24/1, [vel_ned_vera], Discrete-Time Integrator1/1
  Selector28/1 -> Demux19/1
  DATASET NOSTRO1/1(acc) -> [acc_ned_vera], Discrete-Time Integrator/1, acc/1
  Mux25/1 -> Selector30/1
  Digital Clock2/1 -> DATASET NOSTRO1/1(T)
  DATASET NOSTRO1/2(vel) -> Mux24/2
  DATASET NOSTRO1/3(pos) -> Mux25/2
  Demux19/1 -> vel/1
  Demux20/2 -> pos/2
  [acc_ned_vera] -> Subsystem/1(acc_pulita)
  [bias_stima_fd] -> Rate Transition8/1
  Rate Transition8/1 -> Sum2/2
  Selector32/1 -> To Workspace18/1
  Selector33/1 -> To Workspace21/1
  [Rt] -> MATLAB Function/1(Rt)
  Data Type Conversion87/1 -> MATLAB Function1/2(acc_body_sporca), Rate Transition16/1
  [Rt_fd] -> MATLAB Function1/1(Rt)
  Sum1/1 -> ACC_DOPO_AHRS_NED COMPENSATO DI GRAVITA'1/1, [acc_ned_AHRS_fd]
  MATLAB Function1/1(acc_ned) -> Sum1/1
  Data Type Conversion49/1 -> Sum1/2
  gravity2/1 -> Data Type Conversion49/1
  gravity3/1 -> Data Type Conversion50/1
  Sum4/1 -> [acc_ned_AHRS]
  Data Type Conversion50/1 -> Sum4/2
  MATLAB Function/1(acc_ned) -> Sum4/1
  Rate Transition16/1 -> Sum2/1
  Sum2/1 -> MPU AHRS4/1(ACC)
  [PQR_veri] -> Sum5/1
  Sum5/1 -> Scope1/1, Data Type Conversion89/1
  Random Number/1 -> Sum5/2
  Random Number1/1 -> Sum6/2
  [PQR_veri] -> Sum6/1
  Sum6/1 -> Data Type Conversion46/1, Scope2/1
  Demux21/3 -> MATLAB Function3/1(yaw)
  Discrete-Time Integrator2/1 -> Demux21/1
  Demux21/1 -> Cast To Single/1
  Gain6/1 -> RPY1/1
  Gain7/1 -> RPY1/2
  Gain8/1 -> RPY1/3
  Cast To Single/1 -> Mux26/1, Gain6/1
  Demux21/2 -> Cast To Single4/1
  Cast To Single4/1 -> Mux26/2, Gain7/1
  MATLAB Function3/1(yaw_lim) -> Cast To Single5/1
  Cast To Single5/1 -> Mux26/3, Gain8/1
  Rate Transition32/1 -> To Workspace84/1
  [pos_ned_vera] -> Rate Transition30/1
  [RPY_AHRS] -> Gain19/1
  Selector47/1 -> To Workspace78/1
  [RPY_AHRS_fd] -> Gain20/1
  [vel_misura] -> Rate Transition31/1
  b_y5/1 -> To Workspace83/1
  Gain20/1 -> To Workspace88/1
  Rate Transition34/1 -> To Workspace77/1
  Gain18/1 -> To Workspace86/1
  Rate Transition31/1 -> To Workspace74/1
  [acc_ned_AHRS_fd] -> Rate Transition32/1
  Gain19/1 -> To Workspace87/1
  [acc_ned_vera] -> Rate Transition34/1
  Selector48/1 -> To Workspace80/1
  b_x5/1 -> To Workspace82/1
  Selector49/1 -> To Workspace81/1
  Selector46/1 -> To Workspace79/1
  b_z5/1 -> To Workspace85/1
  [vel_ned_vera] -> Rate Transition33/1
  [pos_misura] -> Rate Transition35/1
  Rate Transition35/1 -> To Workspace73/1
  Rate Transition30/1 -> To Workspace75/1
  Rate Transition33/1 -> To Workspace76/1
  [x_out_filter_fd] -> Selector49/1, Selector48/1, Selector47/1, Selector46/1
  [prova] -> Gain18/1

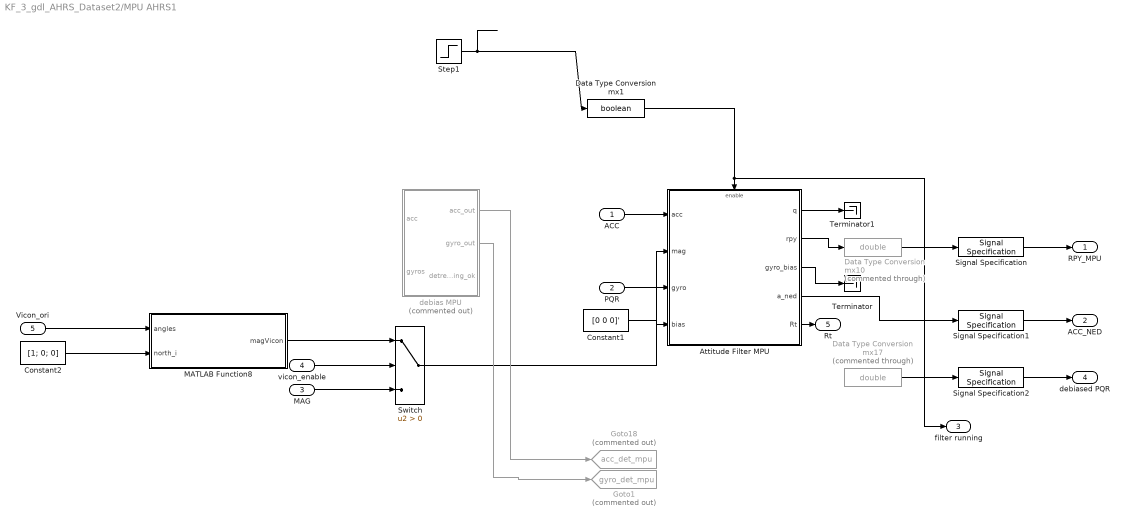
== system KF_3_gdl_AHRS_Dataset2/MPU AHRS1 ==
  ACC : Inport
  PQR : Inport  Port=2
  MAG : Inport  Port=3
  vicon_enable : Inport  Port=4
  Vicon_ori : Inport  Port=5
  Attitude Filter MPU : Subsystem  mask{T=ST}
      mask prompts: T "Sample Time"
  Constant1 : Constant  Value=[0 0 0]'  OutDataTypeStr=single
  Constant2 : Constant  Value=[1; 0; 0]  OutDataTypeStr=single
  Data Type Conversion mx1 : DataTypeConversion  OutDataTypeStr=boolean  RndMeth=Round  SaturateOnIntegerOverflow=on
  Data Type Conversion mx10 : DataTypeConversion  Commented=through  OutDataTypeStr=double  RndMeth=Round  SaturateOnIntegerOverflow=on
  Data Type Conversion mx17 : DataTypeConversion  Commented=through  OutDataTypeStr=double  RndMeth=Round  SaturateOnIntegerOverflow=on
  Goto1 : Goto  Commented=on  GotoTag=gyro_det_mpu  TagVisibility=global
  Goto18 : Goto  Commented=on  GotoTag=acc_det_mpu  TagVisibility=global
  MATLAB Function8 : MATLAB Function  TreatAsAtomicUnit=on
  Signal Specification : SignalSpecification  OutDataTypeStr=single
  Signal Specification1 : SignalSpecification  OutDataTypeStr=single
  Signal Specification2 : SignalSpecification  OutDataTypeStr=single
  Step1 : Step  Time=11  SampleTime=ST
  Switch : Switch  Criteria=u2 > Threshold
  Terminator : Terminator
  Terminator1 : Terminator
  debias MPU : Subsystem  Commented=on
  RPY_MPU : Outport
  ACC_NED : Outport  Port=2
  filter running : Outport  Port=3
  debiased PQR : Outport  Port=4
  Rt : Outport  Port=5
  wires:
  Constant1/1 -> Attitude Filter MPU/4(bias)
  Attitude Filter MPU/2(rpy) -> Data Type Conversion mx10/1
  Switch/1 -> Attitude Filter MPU/2(mag)
  debias MPU/1(acc_out) -> Goto18/1
  debias MPU/2(gyro_out) -> Goto1/1
  Attitude Filter MPU/4(a_ned) -> Signal Specification1/1
  Data Type Conversion mx10/1 -> Signal Specification/1
  Data Type Conversion mx17/1 -> Signal Specification2/1
  Attitude Filter MPU/3(gyro_bias) -> Terminator/1
  Attitude Filter MPU/1(q) -> Terminator1/1
  Signal Specification/1 -> RPY_MPU/1
  Signal Specification1/1 -> ACC_NED/1
  Signal Specification2/1 -> debiased PQR/1
  MAG/1 -> Switch/3
  vicon_enable/1 -> Switch/2
  Vicon_ori/1 -> MATLAB Function8/1(angles)
  Constant2/1 -> MATLAB Function8/2(north_i)
  MATLAB Function8/1(magVicon) -> Switch/1
  Attitude Filter MPU/5(Rt) -> Rt/1
  Step1/1 -> Data Type Conversion mx1/1
  ACC/1 -> Attitude Filter MPU/1(acc)
  PQR/1 -> Attitude Filter MPU/3(gyro)
  Data Type Conversion mx1/1 -> filter running/1, Attitude Filter MPU/Enable

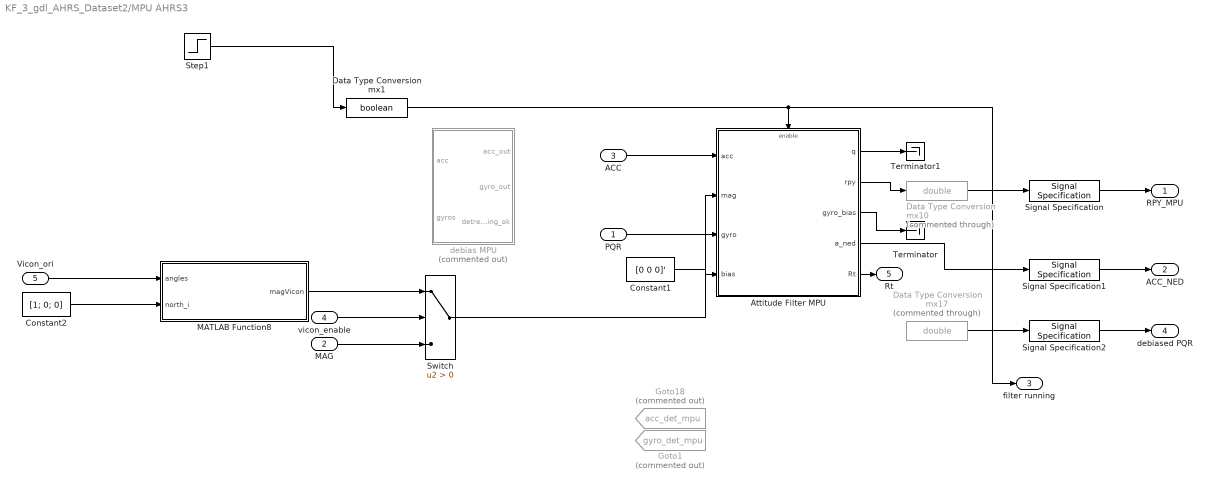
== system KF_3_gdl_AHRS_Dataset2/MPU AHRS3 ==
  PQR : Inport
  MAG : Inport  Port=2
  ACC : Inport  Port=3
  vicon_enable : Inport  Port=4
  Vicon_ori : Inport  Port=5
  Attitude Filter MPU : Subsystem  mask{T=ST}
      mask prompts: T "Sample Time"
  Constant1 : Constant  Value=[0 0 0]'  OutDataTypeStr=single
  Constant2 : Constant  Value=[1; 0; 0]  OutDataTypeStr=single
  Data Type Conversion mx1 : DataTypeConversion  OutDataTypeStr=boolean  RndMeth=Round  SaturateOnIntegerOverflow=on
  Data Type Conversion mx10 : DataTypeConversion  Commented=through  OutDataTypeStr=double  RndMeth=Round  SaturateOnIntegerOverflow=on
  Data Type Conversion mx17 : DataTypeConversion  Commented=through  OutDataTypeStr=double  RndMeth=Round  SaturateOnIntegerOverflow=on
  Goto1 : Goto  Commented=on  GotoTag=gyro_det_mpu  TagVisibility=global
  Goto18 : Goto  Commented=on  GotoTag=acc_det_mpu  TagVisibility=global
  MATLAB Function8 : MATLAB Function  TreatAsAtomicUnit=on
  Signal Specification : SignalSpecification  OutDataTypeStr=single
  Signal Specification1 : SignalSpecification  OutDataTypeStr=single
  Signal Specification2 : SignalSpecification  OutDataTypeStr=single
  Step1 : Step  Time=11  SampleTime=ST
  Switch : Switch  Criteria=u2 > Threshold
  Terminator : Terminator
  Terminator1 : Terminator
  debias MPU : Subsystem  Commented=on
  RPY_MPU : Outport
  ACC_NED : Outport  Port=2
  filter running : Outport  Port=3
  debiased PQR : Outport  Port=4
  Rt : Outport  Port=5
  wires:
  Constant1/1 -> Attitude Filter MPU/4(bias)
  Attitude Filter MPU/2(rpy) -> Data Type Conversion mx10/1
  Switch/1 -> Attitude Filter MPU/2(mag)
  Attitude Filter MPU/4(a_ned) -> Signal Specification1/1
  Data Type Conversion mx10/1 -> Signal Specification/1
  Data Type Conversion mx17/1 -> Signal Specification2/1
  Attitude Filter MPU/3(gyro_bias) -> Terminator/1
  Attitude Filter MPU/1(q) -> Terminator1/1
  Signal Specification/1 -> RPY_MPU/1
  Signal Specification1/1 -> ACC_NED/1
  Signal Specification2/1 -> debiased PQR/1
  MAG/1 -> Switch/3
  vicon_enable/1 -> Switch/2
  Vicon_ori/1 -> MATLAB Function8/1(angles)
  Constant2/1 -> MATLAB Function8/2(north_i)
  MATLAB Function8/1(magVicon) -> Switch/1
  Attitude Filter MPU/5(Rt) -> Rt/1
  Step1/1 -> Data Type Conversion mx1/1
  Data Type Conversion mx1/1 -> filter running/1, Attitude Filter MPU/Enable
  ACC/1 -> Attitude Filter MPU/1(acc)
  PQR/1 -> Attitude Filter MPU/3(gyro)

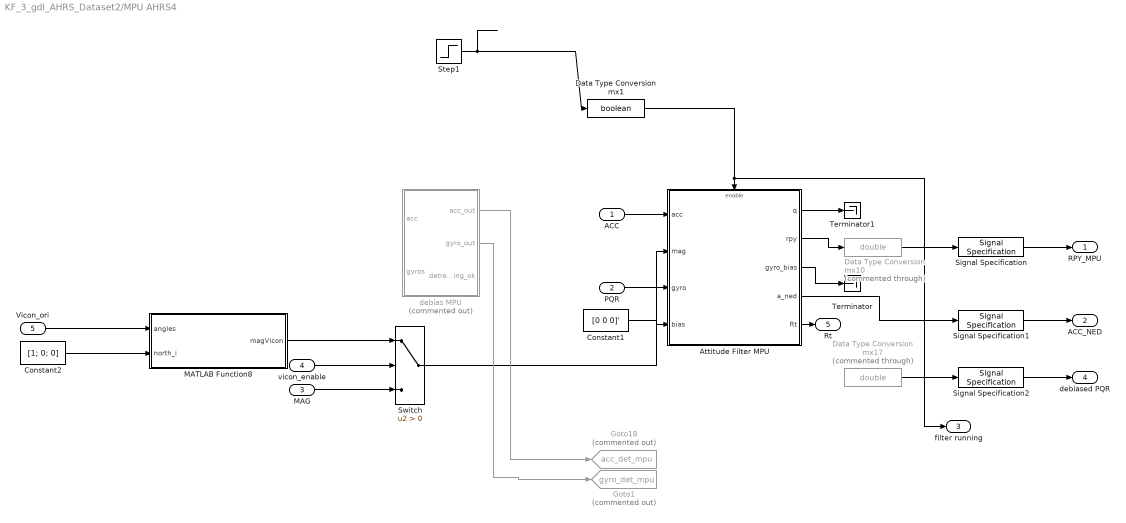
== system KF_3_gdl_AHRS_Dataset2/MPU AHRS4 ==
  ACC : Inport
  PQR : Inport  Port=2
  MAG : Inport  Port=3
  vicon_enable : Inport  Port=4
  Vicon_ori : Inport  Port=5
  Attitude Filter MPU : Subsystem  mask{T=ST}
      mask prompts: T "Sample Time"
  Constant1 : Constant  Value=[0 0 0]'  OutDataTypeStr=single
  Constant2 : Constant  Value=[1; 0; 0]  OutDataTypeStr=single
  Data Type Conversion mx1 : DataTypeConversion  OutDataTypeStr=boolean  RndMeth=Round  SaturateOnIntegerOverflow=on
  Data Type Conversion mx10 : DataTypeConversion  Commented=through  OutDataTypeStr=double  RndMeth=Round  SaturateOnIntegerOverflow=on
  Data Type Conversion mx17 : DataTypeConversion  Commented=through  OutDataTypeStr=double  RndMeth=Round  SaturateOnIntegerOverflow=on
  Goto1 : Goto  Commented=on  GotoTag=gyro_det_mpu  TagVisibility=global
  Goto18 : Goto  Commented=on  GotoTag=acc_det_mpu  TagVisibility=global
  MATLAB Function8 : MATLAB Function  TreatAsAtomicUnit=on
  Signal Specification : SignalSpecification  OutDataTypeStr=single
  Signal Specification1 : SignalSpecification  OutDataTypeStr=single
  Signal Specification2 : SignalSpecification  OutDataTypeStr=single
  Step1 : Step  Time=11  SampleTime=ST
  Switch : Switch  Criteria=u2 > Threshold
  Terminator : Terminator
  Terminator1 : Terminator
  debias MPU : Subsystem  Commented=on
  RPY_MPU : Outport
  ACC_NED : Outport  Port=2
  filter running : Outport  Port=3
  debiased PQR : Outport  Port=4
  Rt : Outport  Port=5
  wires:
  Constant1/1 -> Attitude Filter MPU/4(bias)
  Attitude Filter MPU/2(rpy) -> Data Type Conversion mx10/1
  Switch/1 -> Attitude Filter MPU/2(mag)
  debias MPU/1(acc_out) -> Goto18/1
  debias MPU/2(gyro_out) -> Goto1/1
  Attitude Filter MPU/4(a_ned) -> Signal Specification1/1
  Data Type Conversion mx10/1 -> Signal Specification/1
  Data Type Conversion mx17/1 -> Signal Specification2/1
  Attitude Filter MPU/3(gyro_bias) -> Terminator/1
  Attitude Filter MPU/1(q) -> Terminator1/1
  Signal Specification/1 -> RPY_MPU/1
  Signal Specification1/1 -> ACC_NED/1
  Signal Specification2/1 -> debiased PQR/1
  MAG/1 -> Switch/3
  vicon_enable/1 -> Switch/2
  Vicon_ori/1 -> MATLAB Function8/1(angles)
  Constant2/1 -> MATLAB Function8/2(north_i)
  MATLAB Function8/1(magVicon) -> Switch/1
  Attitude Filter MPU/5(Rt) -> Rt/1
  Step1/1 -> Data Type Conversion mx1/1
  ACC/1 -> Attitude Filter MPU/1(acc)
  PQR/1 -> Attitude Filter MPU/3(gyro)
  Data Type Conversion mx1/1 -> filter running/1, Attitude Filter MPU/Enable

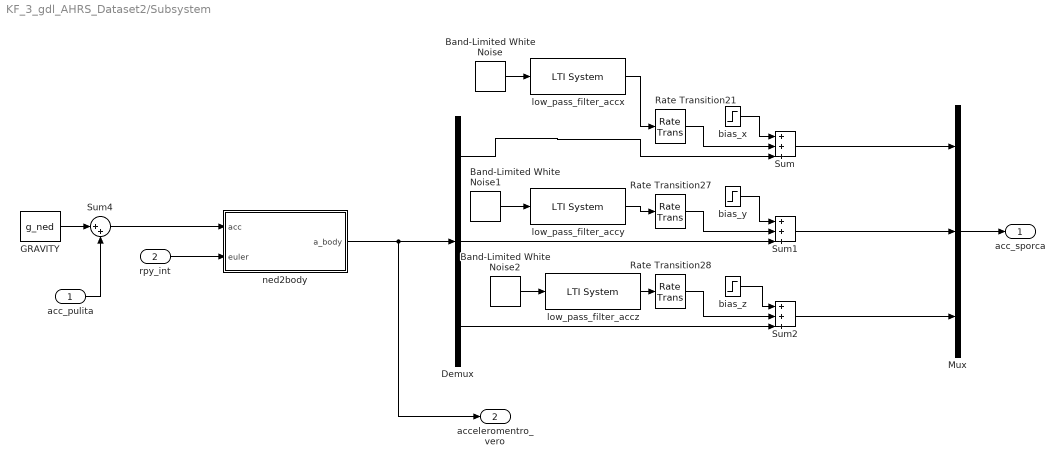
== system KF_3_gdl_AHRS_Dataset2/Subsystem ==
  acc_pulita : Inport
  rpy_int : Inport  Port=2
  Band-Limited White Noise : simulink/Sources/Band-Limited White Noise  Cov=noise_gain  Ts=T_50  seed=[23341]
  Band-Limited White Noise1 : simulink/Sources/Band-Limited White Noise  Cov=noise_gain  Ts=T_50  seed=[23381]
  Band-Limited White Noise2 : simulink/Sources/Band-Limited White Noise  Cov=noise_gain  Ts=T_50  seed=[23741]
  Demux : Demux  Outputs=3
  GRAVITY : Constant  Value=g_ned
  Mux : Mux  Inputs=3
  Rate Transition21 : RateTransition  OutPortSampleTime=1/50
  Rate Transition27 : RateTransition  OutPortSampleTime=1/50
  Rate Transition28 : RateTransition  OutPortSampleTime=1/50
  Sum : Sum  Inputs=|+|+|+
  Sum1 : Sum  Inputs=|+|+|+
  Sum2 : Sum  Inputs=|+|+|+
  Sum4 : Sum  Inputs=|++
  bias_x : Step  Time=11.02  After=bj_x  SampleTime=1/50
  bias_y : Step  Time=11.02  After=bj_y  SampleTime=1/50
  bias_z : Step  Time=11.02  After=bj_z  SampleTime=1/50
  low_pass_filter_accx : cstblocks/LTI System  sys=filter_acc  IC=[]
  low_pass_filter_accy : cstblocks/LTI System  sys=filter_acc  IC=[]
  low_pass_filter_accz : cstblocks/LTI System  sys=filter_acc  IC=[]
  ned2body : MATLAB Function  TreatAsAtomicUnit=on
  acc_sporca : Outport
  acceleromentro_vero : Outport  Port=2
  wires:
  Band-Limited White Noise2/1 -> low_pass_filter_accz/1
  Band-Limited White Noise/1 -> low_pass_filter_accx/1
  Band-Limited White Noise1/1 -> low_pass_filter_accy/1
  Demux/1 -> Sum/3
  bias_x/1 -> Sum/1
  bias_y/1 -> Sum1/1
  bias_z/1 -> Sum2/1
  Mux/1 -> acc_sporca/1
  Sum/1 -> Mux/1
  Sum1/1 -> Mux/2
  Sum2/1 -> Mux/3
  ned2body/1(a_body) -> Demux/1, acceleromentro_vero/1
  rpy_int/1 -> ned2body/2(euler)
  Rate Transition21/1 -> Sum/2
  Rate Transition27/1 -> Sum1/2
  Rate Transition28/1 -> Sum2/2
  acc_pulita/1 -> Sum4/2
  GRAVITY/1 -> Sum4/1
  Sum4/1 -> ned2body/1(acc)
  low_pass_filter_accx/1 -> Rate Transition21/1
  low_pass_filter_accz/1 -> Rate Transition28/1
  low_pass_filter_accy/1 -> Rate Transition27/1
  Demux/2 -> Sum1/3
  Demux/3 -> Sum2/3

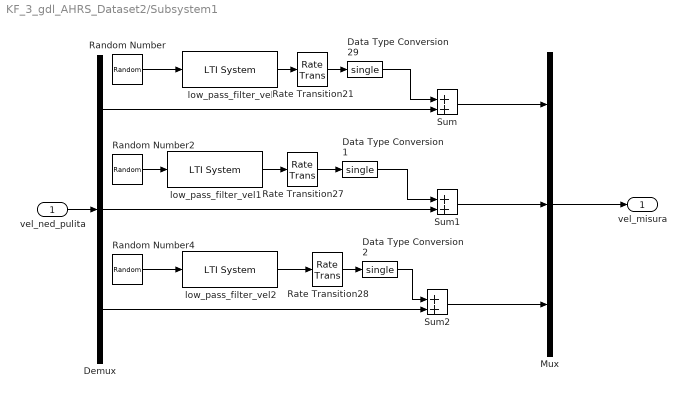
== system KF_3_gdl_AHRS_Dataset2/Subsystem1 ==
  vel_ned_pulita : Inport
  Data Type Conversion1 : DataTypeConversion  OutDataTypeStr=single
  Data Type Conversion2 : DataTypeConversion  OutDataTypeStr=single
  Data Type Conversion29 : DataTypeConversion  OutDataTypeStr=single
  Demux : Demux  Outputs=3
  Mux : Mux  Inputs=3
  Random Number : RandomNumber  Variance=var_v_x*5  SampleTime=0.02
  Random Number2 : RandomNumber  Variance=var_v_y*10  Seed=1  SampleTime=0.02
  Random Number4 : RandomNumber  Variance=var_v_z*5  Seed=2  SampleTime=0.02
  Rate Transition21 : RateTransition  OutPortSampleTime=1/50
  Rate Transition27 : RateTransition  OutPortSampleTime=1/50
  Rate Transition28 : RateTransition  OutPortSampleTime=1/50
  Sum : Sum  Inputs=|+|+
  Sum1 : Sum  Inputs=|+|+
  Sum2 : Sum  Inputs=|+|+
  low_pass_filter_vel : cstblocks/LTI System  sys=filter_vel  IC=[]
  low_pass_filter_vel1 : cstblocks/LTI System  sys=filter_vel  IC=[]
  low_pass_filter_vel2 : cstblocks/LTI System  sys=filter_vel  IC=[]
  vel_misura : Outport
  wires:
  low_pass_filter_vel/1 -> Rate Transition21/1
  Random Number2/1 -> low_pass_filter_vel1/1
  Random Number4/1 -> low_pass_filter_vel2/1
  low_pass_filter_vel1/1 -> Rate Transition27/1
  low_pass_filter_vel2/1 -> Rate Transition28/1
  Random Number/1 -> low_pass_filter_vel/1
  vel_ned_pulita/1 -> Demux/1
  Demux/1 -> Sum/2
  Demux/2 -> Sum1/2
  Demux/3 -> Sum2/2
  Sum2/1 -> Mux/3
  Sum1/1 -> Mux/2
  Sum/1 -> Mux/1
  Mux/1 -> vel_misura/1
  Rate Transition21/1 -> Data Type Conversion29/1
  Data Type Conversion29/1 -> Sum/1
  Rate Transition27/1 -> Data Type Conversion1/1
  Data Type Conversion1/1 -> Sum1/1
  Rate Transition28/1 -> Data Type Conversion2/1
  Data Type Conversion2/1 -> Sum2/1

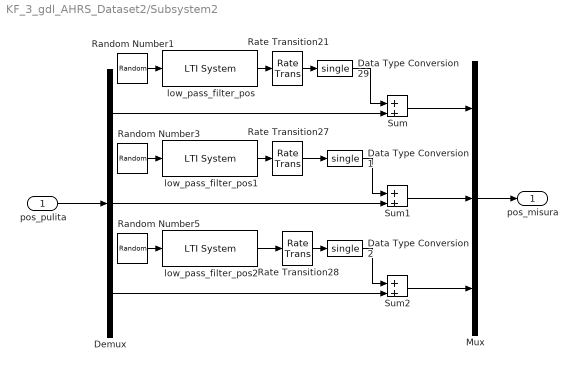
== system KF_3_gdl_AHRS_Dataset2/Subsystem2 ==
  pos_pulita : Inport
  Data Type Conversion1 : DataTypeConversion  OutDataTypeStr=single
  Data Type Conversion2 : DataTypeConversion  OutDataTypeStr=single
  Data Type Conversion29 : DataTypeConversion  OutDataTypeStr=single
  Demux : Demux  Outputs=3
  Mux : Mux  Inputs=3
  Random Number1 : RandomNumber  Variance=var_p_x  Seed=3  SampleTime=1/200
  Random Number3 : RandomNumber  Variance=var_p_y  Seed=85  SampleTime=1/200
  Random Number5 : RandomNumber  Variance=var_p_z  Seed=57  SampleTime=1/200
  Rate Transition21 : RateTransition  OutPortSampleTime=1/50
  Rate Transition27 : RateTransition  OutPortSampleTime=1/50
  Rate Transition28 : RateTransition  OutPortSampleTime=1/50
  Sum : Sum  Inputs=|+|+
  Sum1 : Sum  Inputs=|+|+
  Sum2 : Sum  Inputs=|+|+
  low_pass_filter_pos : cstblocks/LTI System  sys=filter_pos*10  IC=[]
  low_pass_filter_pos1 : cstblocks/LTI System  sys=filter_pos*10  IC=[]
  low_pass_filter_pos2 : cstblocks/LTI System  sys=filter_pos_Z*10  IC=[]
  pos_misura : Outport
  wires:
  low_pass_filter_pos/1 -> Rate Transition21/1
  Random Number5/1 -> low_pass_filter_pos2/1
  Random Number3/1 -> low_pass_filter_pos1/1
  low_pass_filter_pos2/1 -> Rate Transition28/1
  low_pass_filter_pos1/1 -> Rate Transition27/1
  Random Number1/1 -> low_pass_filter_pos/1
  pos_pulita/1 -> Demux/1
  Demux/1 -> Sum/2
  Demux/2 -> Sum1/2
  Demux/3 -> Sum2/2
  Sum1/1 -> Mux/2
  Sum/1 -> Mux/1
  Sum2/1 -> Mux/3
  Mux/1 -> pos_misura/1
  Rate Transition21/1 -> Data Type Conversion29/1
  Data Type Conversion29/1 -> Sum/1
  Rate Transition27/1 -> Data Type Conversion1/1
  Data Type Conversion1/1 -> Sum1/1
  Rate Transition28/1 -> Data Type Conversion2/1
  Data Type Conversion2/1 -> Sum2/1

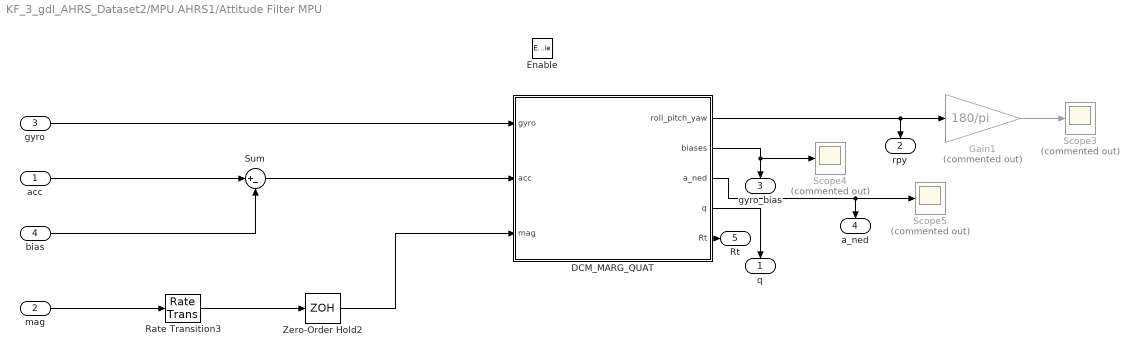
== system KF_3_gdl_AHRS_Dataset2/MPU AHRS1/Attitude Filter MPU ==
  acc : Inport
  mag : Inport  Port=2
  gyro : Inport  Port=3
  bias : Inport  Port=4
  Enable : EnablePort  StatesWhenEnabling=reset
  DCM_MARG_QUAT : Subsystem  mask{Kp=0.15, Ki=0, tau=40, T=T}
      mask prompts: Kp "Proportional Gain"; Ki "Integral Gain"; tau "Biases Time Constant"; T "Sample Time"
  Gain1 : Gain  Commented=on  Gain=180/pi
  Rate Transition3 : RateTransition  Deterministic=off
  Scope3 : Scope  Commented=on
  Scope4 : Scope  Commented=on
  Scope5 : Scope  Commented=on
  Sum : Sum  Inputs=|+-
  Zero-Order Hold2 : ZeroOrderHold  SampleTime=T
  q : Outport  PortDimensions=4  InitialOutput=[1 0 0 0]'
  rpy : Outport  Port=2  PortDimensions=3  InitialOutput=[0 0 0]'
  gyro_bias : Outport  Port=3  PortDimensions=3  InitialOutput=[0 0 0]'
  a_ned : Outport  Port=4  InitialOutput=[0 0 0]'
  Rt : Outport  Port=5
  wires:
  Rate Transition3/1 -> Zero-Order Hold2/1
  Zero-Order Hold2/1 -> DCM_MARG_QUAT/3(mag)
  DCM_MARG_QUAT/4(q) -> q/1
  bias/1 -> Sum/2
  Sum/1 -> DCM_MARG_QUAT/2(acc)
  acc/1 -> Sum/1
  DCM_MARG_QUAT/3(a_ned) -> a_ned/1, Scope5/1
  DCM_MARG_QUAT/1(roll_pitch_yaw) -> rpy/1, Gain1/1
  mag/1 -> Rate Transition3/1
  gyro/1 -> DCM_MARG_QUAT/1(gyro)
  DCM_MARG_QUAT/2(biases) -> gyro_bias/1, Scope4/1
  Gain1/1 -> Scope3/1
  DCM_MARG_QUAT/5(Rt) -> Rt/1
